simulink model "gm_mpu6050_interfaceasdf"  (R2017a)
settings: Solver=FixedStepDiscrete  StartTime=0.0  StopTime=inf  RelTol=1e-3  EnableMultiTasking=on
PostLoadFcn:
  | ChipSelect = 1;  % choose I2C comms
  | AddressAlt = 0;  % use default address
  | 
  | if AddressAlt == 1
  | % b1101001 (pin AD0 is logic high).
  | SlvAddr = uint8(bin2dec('1101001'));  % ADDR ALT = 1
  | else
  | % b1101000 (pin AD0 is logic low)
  | SlvAddr = uint8(bin2dec('1101000'));  % ADDR ALT = 0
  | end
  | SlvAddr = uint8(hex2dec('68'));
  | 
  | 
  | % 0x3B 59 ACCEL_XOUT[15:8]
  | % 0x3C 60 ACCEL_XOUT[7:0]
  | % 0x3D 61 ACCEL_YOUT[15:8]
  | % 0x3E 62 ACCEL_YOUT[7:0]
  | % 0x3F 63 ACCEL_ZOUT[15:8]
  | % 0x40 64 ACCEL_ZOUT[7:0]
  | 
  | AccelXRegAddr = uint8(hex2dec('3B'));
  | AccelYRegAddr = uint8(hex2dec('3D'));
  | AccelZRegAddr = uint8(hex2dec('3F'));
  | 
  | % 0x43 67 GYRO_XOUT[15:8]
  | % 0x44 68 GYRO_XOUT[7:0]
  | % 0x45 69 GYRO_YOUT[15:8]
  | % 0x46 70 GYRO_YOUT[7:0]
  | % 0x47 71 GYRO_ZOUT[15:8]
  | % 0x48 72 GYRO_ZOUT[7:0]
  | 
  | GyroXRegAddr = uint8(hex2dec('43'));
  | GyroYRegAddr = uint8(hex2dec('45'));
  | GyroZRegAddr = uint8(hex2dec('47'));
  | 
  | deviceAddr = fi(SlvAddr,0,7,0);
  | 
  | powerRegAddr = uint8(hex2dec('6B'));
  | powerRegData = bin2dec('10000001');
undefined symbols (not defined in the file): AXI4, Lite
libraries: axiinterfacelib x10
settings Model: SimulationMode=external  Creator=skuznick  LastModifiedBy=mini
settings SolverCC: EnableConcurrentExecution=on  ConcurrentTasks=on  PositivePriorityOrder=on
settings DataIOCC: SaveOutput=off  SaveTime=off
settings OptimizationCC: BlockReduction=off  ConditionallyExecuteInputs=off  PassReuseOutputArgsAs=Individual arguments  MaxStackSize=64
settings DebuggingCC: AlgebraicLoopMsg=error  SingleTaskRateTransMsg=error  ParameterTunabilityLossMsg=error
settings HardwareCC: ProdBitPerPointer=32  ProdBitPerSizeT=32  ProdBitPerPtrDiffT=32  ProdLargestAtomicInteger=Long  ProdLargestAtomicFloat=Double  ProdWordSize=32  ProdHWDeviceType=ARM Compatible->ARM Cortex  TargetEndianess=LittleEndian
settings SFSimCC: MATLABDynamicMemAlloc=off
settings RTWCC: SystemTargetFile=ert.tlc  HardwareBoard=ZedBoard  TLCOptions="-aInlineSetEventsForThisBaseRateFcn=TLC_FALSE -aSuppressMultiTaskScheduler=TLC_FALSE  -aRateBasedStepFcn=0"  TemplateMakefile=ert_default_tmf  Description=Embedded Coder  GenerateReport=on  Toolchain=Xilinx Software Development Kit (SDK)  IncludeHyperlinkInReport=on  LaunchReport=on  GenerateTraceInfo=on  GenerateTraceReport=on  GenerateTraceReportSl=on  GenerateTraceReportSf=on  GenerateTraceReportEml=on
settings CodeAppCC: ForceParamTrailComments=on  IgnoreCustomStorageClasses=off  OperatorAnnotations=on  SimulinkDataObjDesc=on  SFDataObjDesc=on  MATLABFcnDesc=on  InsertBlockDesc=on  MATLABSourceComments=on

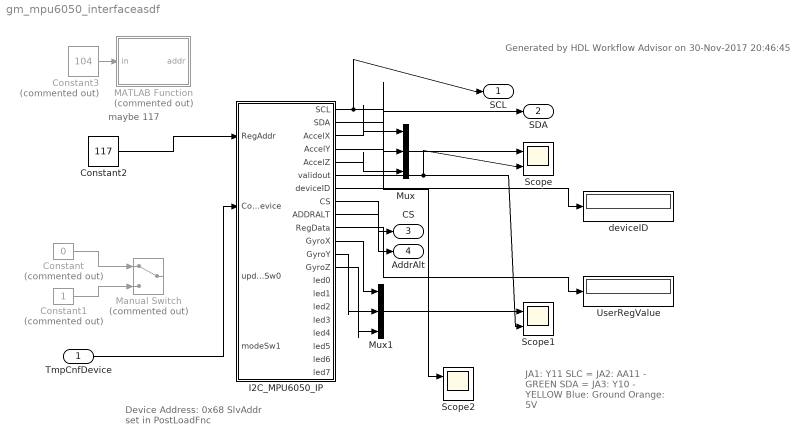
== system gm_mpu6050_interfaceasdf ==
  note: Device Address: 0x68
      | SlvAddr set in PostLoadFnc
  note: JA1: Y11
      | SLC = JA2: AA11 - GREEN
      | SDA = JA3: Y10  - YELLOW
      | Blue: Ground
      | Orange: 5V
  note: maybe 117
  note: Generated by HDL Workflow Advisor on 30-Nov-2017 20:46:45
  TmpCnfDevice : Inport  OutDataTypeStr=boolean
  Constant : Constant  Commented=on  Value=0  OutDataTypeStr=boolean  SampleTime=-1
  Constant1 : Constant  Commented=on  OutDataTypeStr=boolean  SampleTime=-1
  Constant2 : Constant  Value=117  OutDataTypeStr=uint8  SampleTime=-1
  Constant3 : Constant  Commented=on  Value=104  OutDataTypeStr=uint8  SampleTime=-1
  I2C_MPU6050_IP : Subsystem  TreatAsAtomicUnit=on  mask(AXI4-Lite/AXI4 Interface){}
      mask help:
      | This is an automatically generated subsystem block.
      | This contains the AXI interface blocks that communicate with the ADXL345_ip IPCore generated from mpu6050/I2C_MPU6050_IP subsystem.
      mask Display: disp(sprintf('Xilinx Zynq \nAXI Interface'));
  MATLAB Function : MATLAB Function  Commented=on  TreatAsAtomicUnit=on
  Manual Switch : ManualSwitch  Commented=on
  Mux : Mux  Inputs=3
  Mux1 : Mux  Inputs=3
  Scope : Scope  NumInputPorts=2
  Scope1 : Scope  NumInputPorts=2
  Scope2 : Scope  NumInputPorts=2
  UserRegValue : Display
  deviceID : Display
  SCL : Outport
  SDA : Outport  Port=2
  CS : Outport  Port=3
  AddrAlt : Outport  Port=4
  wires:
  Constant3/1 -> MATLAB Function/1(in)
  TmpCnfDevice/1 -> I2C_MPU6050_IP/2(ConfigDevice)
  I2C_MPU6050_IP/6(validout) -> Scope1/2, Scope/2
  I2C_MPU6050_IP/12(GyroY) -> Mux1/2
  I2C_MPU6050_IP/11(GyroX) -> Mux1/1
  I2C_MPU6050_IP/13(GyroZ) -> Mux1/3
  Mux1/1 -> Scope1/1
  Constant2/1 -> I2C_MPU6050_IP/1(RegAddr)
  Constant1/1 -> Manual Switch/2
  Constant/1 -> Manual Switch/1
  Mux/1 -> Scope/1
  I2C_MPU6050_IP/10(RegData) -> UserRegValue/1
  I2C_MPU6050_IP/7(deviceID) -> deviceID/1
  I2C_MPU6050_IP/5(AccelZ) -> Mux/3
  I2C_MPU6050_IP/3(AccelX) -> Mux/1
  I2C_MPU6050_IP/4(AccelY) -> Mux/2
  I2C_MPU6050_IP/9(ADDRALT) -> AddrAlt/1
  I2C_MPU6050_IP/8(CS) -> CS/1
  I2C_MPU6050_IP/1(SCL) -> SCL/1, Scope2/1
  I2C_MPU6050_IP/2(SDA) -> SDA/1

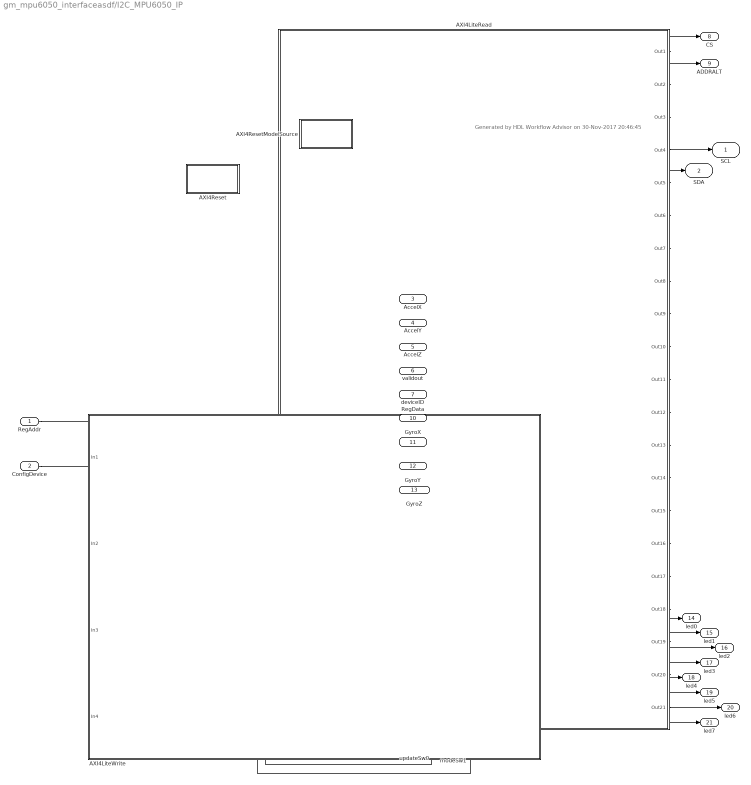
== system gm_mpu6050_interfaceasdf/I2C_MPU6050_IP ==
  note: Generated by HDL Workflow Advisor on 30-Nov-2017 20:46:45
  RegAddr : Inport
  ConfigDevice : Inport  Port=2
  updateSw0 : Inport  Port=3  OutDataTypeStr=boolean
  modeSw1 : Inport  Port=4  OutDataTypeStr=boolean
  AXI4LiteRead : Subsystem  Priority=10
  AXI4LiteWrite : Subsystem  Priority=1
  AXI4Reset : Subsystem  mask(System Start){ShowInLibBrowser=0}
      mask prompts: ShowInLibBrowser "Simulink:masks:CustCodeMaskParam1_MP"
      settings: CopyFcn=cccopyfcn(gcb)  OpenFcn=ccopenfcn('System Start Function')
      mask Help: eval('feval(''rtwprivate'',''rtwhelpview'',''rtw_sys_start_block'')');
      mask Display: disp('System\nStart');
  AXI4ResetModelSource : Subsystem  mask(Model Source){ShowInLibBrowser=0}
      mask prompts: ShowInLibBrowser "Simulink:masks:CustCodeMaskParam1_MP"
      settings: CopyFcn=cccopyfcn(gcb)  OpenFcn=ccopenfcn('Model Source')
      mask Help: eval('feval(''rtwprivate'',''rtwhelpview'',''rtw_model_source_block'')');
      mask Display: disp('Model\nSource');
  SCL : Outport
  SDA : Outport  Port=2
  AccelX : Outport  Port=3
  AccelY : Outport  Port=4
  AccelZ : Outport  Port=5
  validout : Outport  Port=6
  deviceID : Outport  Port=7
  CS : Outport  Port=8
  ADDRALT : Outport  Port=9
  RegData : Outport  Port=10
  GyroX : Outport  Port=11
  GyroY : Outport  Port=12
  GyroZ : Outport  Port=13
  led0 : Outport  Port=14  OutDataTypeStr=boolean
  led1 : Outport  Port=15  OutDataTypeStr=boolean
  led2 : Outport  Port=16  OutDataTypeStr=boolean
  led3 : Outport  Port=17  OutDataTypeStr=boolean
  led4 : Outport  Port=18  OutDataTypeStr=boolean
  led5 : Outport  Port=19  OutDataTypeStr=boolean
  led6 : Outport  Port=20  OutDataTypeStr=boolean
  led7 : Outport  Port=21  OutDataTypeStr=boolean
  wires:
  RegAddr/1 -> AXI4LiteWrite/1(In1)
  ConfigDevice/1 -> AXI4LiteWrite/2(In2)
  updateSw0/1 -> AXI4LiteWrite/3(In3)
  modeSw1/1 -> AXI4LiteWrite/4(In4)
  AXI4LiteRead/1(Out1) -> CS/1
  AXI4LiteRead/2(Out2) -> ADDRALT/1
  AXI4LiteRead/3(Out3) -> SCL/1
  AXI4LiteRead/4(Out4) -> SDA/1
  AXI4LiteRead/5(Out5) -> AccelX/1
  AXI4LiteRead/6(Out6) -> AccelY/1
  AXI4LiteRead/7(Out7) -> AccelZ/1
  AXI4LiteRead/8(Out8) -> validout/1
  AXI4LiteRead/9(Out9) -> deviceID/1
  AXI4LiteRead/10(Out10) -> RegData/1
  AXI4LiteRead/11(Out11) -> GyroX/1
  AXI4LiteRead/12(Out12) -> GyroY/1
  AXI4LiteRead/13(Out13) -> GyroZ/1
  AXI4LiteRead/14(Out14) -> led0/1
  AXI4LiteRead/15(Out15) -> led1/1
  AXI4LiteRead/16(Out16) -> led2/1
  AXI4LiteRead/17(Out17) -> led3/1
  AXI4LiteRead/18(Out18) -> led4/1
  AXI4LiteRead/19(Out19) -> led5/1
  AXI4LiteRead/20(Out20) -> led6/1
  AXI4LiteRead/21(Out21) -> led7/1

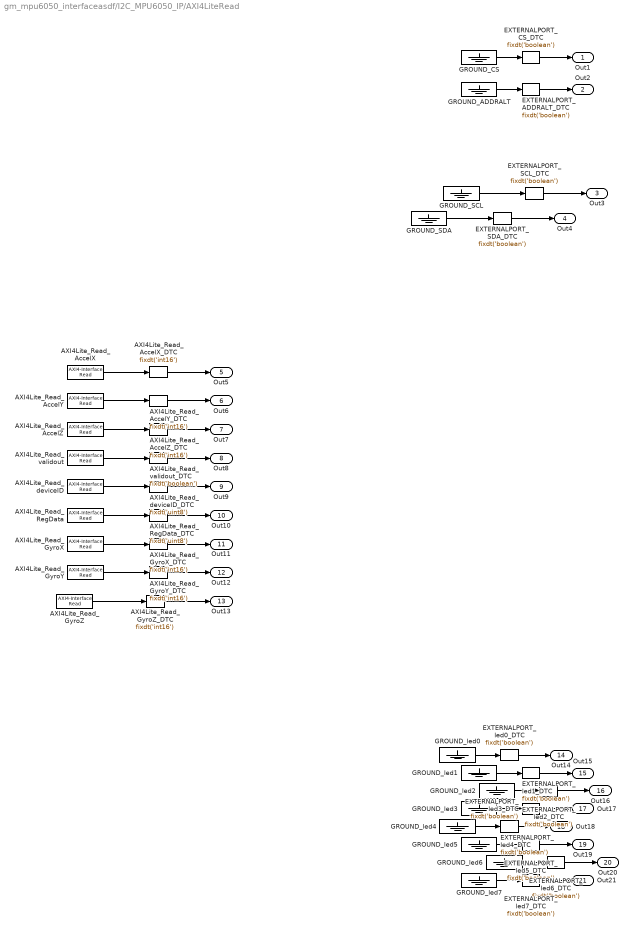
== system gm_mpu6050_interfaceasdf/I2C_MPU6050_IP/AXI4LiteRead ==
  AXI4Lite_Read_AccelX : axiinterfacelib/AXI4-Interface Read  Priority=4  AXIInterfaceType=AXI4-Lite  DeviceName=/dev/mwipcore  RegisterOffset=hex2dec('108')  DataLength=1  DataType=uint32  SampleTime=-1  blockPlatform=ZYNQ  SimulateUsing=Interpreted Execution
      settings: SourceProductName=Embedded Coder Support Package for Xilinx Zynq-7000 Platform  SourceProductBaseCode=ECZYNQ7000
  AXI4Lite_Read_AccelX_DTC : DataTypeConversion  OutDataTypeStr=fixdt('int16')  ConvertRealWorld=Stored Integer (SI)
  AXI4Lite_Read_AccelY : axiinterfacelib/AXI4-Interface Read  Priority=5  AXIInterfaceType=AXI4-Lite  DeviceName=/dev/mwipcore  RegisterOffset=hex2dec('10C')  DataLength=1  DataType=uint32  SampleTime=-1  blockPlatform=ZYNQ  SimulateUsing=Interpreted Execution
      settings: SourceProductName=Embedded Coder Support Package for Xilinx Zynq-7000 Platform  SourceProductBaseCode=ECZYNQ7000
  AXI4Lite_Read_AccelY_DTC : DataTypeConversion  OutDataTypeStr=fixdt('int16')  ConvertRealWorld=Stored Integer (SI)
  AXI4Lite_Read_AccelZ : axiinterfacelib/AXI4-Interface Read  Priority=6  AXIInterfaceType=AXI4-Lite  DeviceName=/dev/mwipcore  RegisterOffset=hex2dec('110')  DataLength=1  DataType=uint32  SampleTime=-1  blockPlatform=ZYNQ  SimulateUsing=Interpreted Execution
      settings: SourceProductName=Embedded Coder Support Package for Xilinx Zynq-7000 Platform  SourceProductBaseCode=ECZYNQ7000
  AXI4Lite_Read_AccelZ_DTC : DataTypeConversion  OutDataTypeStr=fixdt('int16')  ConvertRealWorld=Stored Integer (SI)
  AXI4Lite_Read_GyroX : axiinterfacelib/AXI4-Interface Read  Priority=12  AXIInterfaceType=AXI4-Lite  DeviceName=/dev/mwipcore  RegisterOffset=hex2dec('124')  DataLength=1  DataType=uint32  SampleTime=-1  blockPlatform=ZYNQ  SimulateUsing=Interpreted Execution
      settings: SourceProductName=Embedded Coder Support Package for Xilinx Zynq-7000 Platform  SourceProductBaseCode=ECZYNQ7000
  AXI4Lite_Read_GyroX_DTC : DataTypeConversion  OutDataTypeStr=fixdt('int16')  ConvertRealWorld=Stored Integer (SI)
  AXI4Lite_Read_GyroY : axiinterfacelib/AXI4-Interface Read  Priority=13  AXIInterfaceType=AXI4-Lite  DeviceName=/dev/mwipcore  RegisterOffset=hex2dec('128')  DataLength=1  DataType=uint32  SampleTime=-1  blockPlatform=ZYNQ  SimulateUsing=Interpreted Execution
      settings: SourceProductName=Embedded Coder Support Package for Xilinx Zynq-7000 Platform  SourceProductBaseCode=ECZYNQ7000
  AXI4Lite_Read_GyroY_DTC : DataTypeConversion  OutDataTypeStr=fixdt('int16')  ConvertRealWorld=Stored Integer (SI)
  AXI4Lite_Read_GyroZ : axiinterfacelib/AXI4-Interface Read  Priority=14  AXIInterfaceType=AXI4-Lite  DeviceName=/dev/mwipcore  RegisterOffset=hex2dec('12C')  DataLength=1  DataType=uint32  SampleTime=-1  blockPlatform=ZYNQ  SimulateUsing=Interpreted Execution
      settings: SourceProductName=Embedded Coder Support Package for Xilinx Zynq-7000 Platform  SourceProductBaseCode=ECZYNQ7000
  AXI4Lite_Read_GyroZ_DTC : DataTypeConversion  OutDataTypeStr=fixdt('int16')  ConvertRealWorld=Stored Integer (SI)
  AXI4Lite_Read_RegData : axiinterfacelib/AXI4-Interface Read  Priority=11  AXIInterfaceType=AXI4-Lite  DeviceName=/dev/mwipcore  RegisterOffset=hex2dec('120')  DataLength=1  DataType=uint32  SampleTime=-1  blockPlatform=ZYNQ  SimulateUsing=Interpreted Execution
      settings: SourceProductName=Embedded Coder Support Package for Xilinx Zynq-7000 Platform  SourceProductBaseCode=ECZYNQ7000
  AXI4Lite_Read_RegData_DTC : DataTypeConversion  OutDataTypeStr=fixdt('uint8')  ConvertRealWorld=Stored Integer (SI)
  AXI4Lite_Read_deviceID : axiinterfacelib/AXI4-Interface Read  Priority=8  AXIInterfaceType=AXI4-Lite  DeviceName=/dev/mwipcore  RegisterOffset=hex2dec('11C')  DataLength=1  DataType=uint32  SampleTime=-1  blockPlatform=ZYNQ  SimulateUsing=Interpreted Execution
      settings: SourceProductName=Embedded Coder Support Package for Xilinx Zynq-7000 Platform  SourceProductBaseCode=ECZYNQ7000
  AXI4Lite_Read_deviceID_DTC : DataTypeConversion  OutDataTypeStr=fixdt('uint8')  ConvertRealWorld=Stored Integer (SI)
  AXI4Lite_Read_validout : axiinterfacelib/AXI4-Interface Read  Priority=7  AXIInterfaceType=AXI4-Lite  DeviceName=/dev/mwipcore  RegisterOffset=hex2dec('118')  DataLength=1  DataType=uint32  SampleTime=-1  blockPlatform=ZYNQ  SimulateUsing=Interpreted Execution
      settings: SourceProductName=Embedded Coder Support Package for Xilinx Zynq-7000 Platform  SourceProductBaseCode=ECZYNQ7000
  AXI4Lite_Read_validout_DTC : DataTypeConversion  OutDataTypeStr=fixdt('boolean')  ConvertRealWorld=Stored Integer (SI)
  EXTERNALPORT_ADDRALT_DTC : DataTypeConversion  OutDataTypeStr=fixdt('boolean')
  EXTERNALPORT_CS_DTC : DataTypeConversion  OutDataTypeStr=fixdt('boolean')
  EXTERNALPORT_SCL_DTC : DataTypeConversion  OutDataTypeStr=fixdt('boolean')
  EXTERNALPORT_SDA_DTC : DataTypeConversion  OutDataTypeStr=fixdt('boolean')
  EXTERNALPORT_led0_DTC : DataTypeConversion  OutDataTypeStr=fixdt('boolean')
  EXTERNALPORT_led1_DTC : DataTypeConversion  OutDataTypeStr=fixdt('boolean')
  EXTERNALPORT_led2_DTC : DataTypeConversion  OutDataTypeStr=fixdt('boolean')
  EXTERNALPORT_led3_DTC : DataTypeConversion  OutDataTypeStr=fixdt('boolean')
  EXTERNALPORT_led4_DTC : DataTypeConversion  OutDataTypeStr=fixdt('boolean')
  EXTERNALPORT_led5_DTC : DataTypeConversion  OutDataTypeStr=fixdt('boolean')
  EXTERNALPORT_led6_DTC : DataTypeConversion  OutDataTypeStr=fixdt('boolean')
  EXTERNALPORT_led7_DTC : DataTypeConversion  OutDataTypeStr=fixdt('boolean')
  GROUND_ADDRALT : Ground
  GROUND_CS : Ground
  GROUND_SCL : Ground
  GROUND_SDA : Ground
  GROUND_led{0..7} (8 alike) : Ground
  Out1 : Outport
  Out2 : Outport  Port=2
  Out3 : Outport  Port=3
  Out4 : Outport  Port=4
  Out5 : Outport  Port=5
  Out6 : Outport  Port=6
  Out7 : Outport  Port=7
  Out8 : Outport  Port=8
  Out9 : Outport  Port=9
  Out10 : Outport  Port=10
  Out11 : Outport  Port=11
  Out12 : Outport  Port=12
  Out13 : Outport  Port=13
  Out14 : Outport  Port=14
  Out15 : Outport  Port=15
  Out16 : Outport  Port=16
  Out17 : Outport  Port=17
  Out18 : Outport  Port=18
  Out19 : Outport  Port=19
  Out20 : Outport  Port=20
  Out21 : Outport  Port=21
  wires:
  AXI4Lite_Read_RegData/1 -> AXI4Lite_Read_RegData_DTC/1
  AXI4Lite_Read_RegData_DTC/1 -> Out10/1
  AXI4Lite_Read_GyroX/1 -> AXI4Lite_Read_GyroX_DTC/1
  AXI4Lite_Read_GyroX_DTC/1 -> Out11/1
  GROUND_led0/1 -> EXTERNALPORT_led0_DTC/1
  AXI4Lite_Read_GyroZ/1 -> AXI4Lite_Read_GyroZ_DTC/1
  AXI4Lite_Read_GyroZ_DTC/1 -> Out13/1
  GROUND_led1/1 -> EXTERNALPORT_led1_DTC/1
  EXTERNALPORT_led1_DTC/1 -> Out15/1
  EXTERNALPORT_led0_DTC/1 -> Out14/1
  GROUND_led2/1 -> EXTERNALPORT_led2_DTC/1
  EXTERNALPORT_led4_DTC/1 -> Out18/1
  GROUND_led3/1 -> EXTERNALPORT_led3_DTC/1
  EXTERNALPORT_led2_DTC/1 -> Out16/1
  GROUND_led4/1 -> EXTERNALPORT_led4_DTC/1
  EXTERNALPORT_led3_DTC/1 -> Out17/1
  GROUND_led5/1 -> EXTERNALPORT_led5_DTC/1
  EXTERNALPORT_led5_DTC/1 -> Out19/1
  GROUND_led6/1 -> EXTERNALPORT_led6_DTC/1
  EXTERNALPORT_led6_DTC/1 -> Out20/1
  GROUND_led7/1 -> EXTERNALPORT_led7_DTC/1
  EXTERNALPORT_led7_DTC/1 -> Out21/1
  AXI4Lite_Read_AccelZ/1 -> AXI4Lite_Read_AccelZ_DTC/1
  AXI4Lite_Read_AccelZ_DTC/1 -> Out7/1
  AXI4Lite_Read_GyroY/1 -> AXI4Lite_Read_GyroY_DTC/1
  AXI4Lite_Read_GyroY_DTC/1 -> Out12/1
  EXTERNALPORT_CS_DTC/1 -> Out1/1
  AXI4Lite_Read_deviceID_DTC/1 -> Out9/1
  GROUND_CS/1 -> EXTERNALPORT_CS_DTC/1
  GROUND_ADDRALT/1 -> EXTERNALPORT_ADDRALT_DTC/1
  EXTERNALPORT_ADDRALT_DTC/1 -> Out2/1
  EXTERNALPORT_SCL_DTC/1 -> Out3/1
  GROUND_SDA/1 -> EXTERNALPORT_SDA_DTC/1
  GROUND_SCL/1 -> EXTERNALPORT_SCL_DTC/1
  EXTERNALPORT_SDA_DTC/1 -> Out4/1
  AXI4Lite_Read_AccelX/1 -> AXI4Lite_Read_AccelX_DTC/1
  AXI4Lite_Read_AccelX_DTC/1 -> Out5/1
  AXI4Lite_Read_validout_DTC/1 -> Out8/1
  AXI4Lite_Read_deviceID/1 -> AXI4Lite_Read_deviceID_DTC/1
  AXI4Lite_Read_AccelY_DTC/1 -> Out6/1
  AXI4Lite_Read_validout/1 -> AXI4Lite_Read_validout_DTC/1
  AXI4Lite_Read_AccelY/1 -> AXI4Lite_Read_AccelY_DTC/1

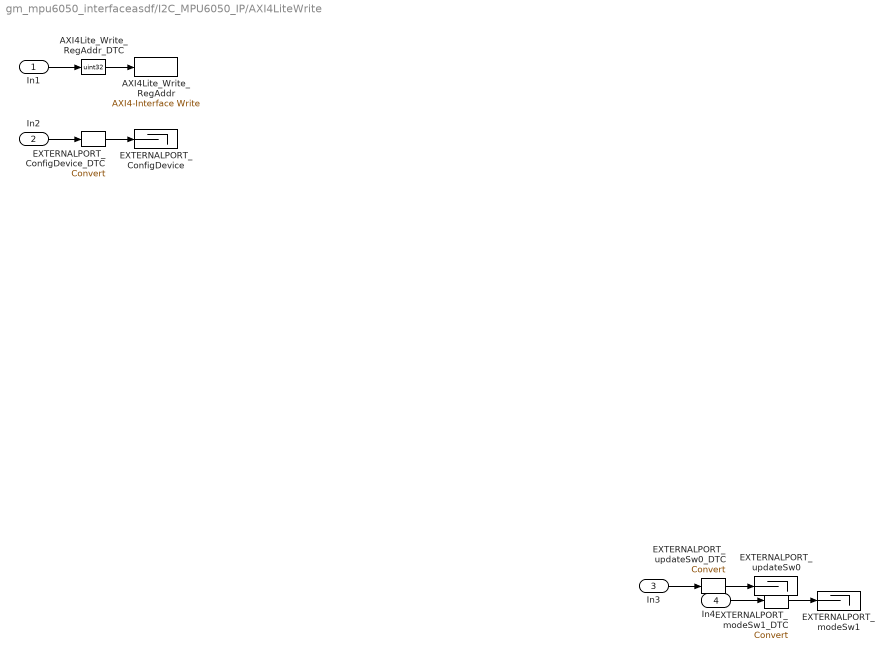
== system gm_mpu6050_interfaceasdf/I2C_MPU6050_IP/AXI4LiteWrite ==
  In1 : Inport
  In2 : Inport  Port=2
  In3 : Inport  Port=3
  In4 : Inport  Port=4
  AXI4Lite_Write_RegAddr : axiinterfacelib/AXI4-Interface Write  Priority=1  AXIInterfaceType=AXI4-Lite  DeviceName=/dev/mwipcore  RegisterOffset=hex2dec('114')  blockPlatform=ZYNQ  SimulateUsing=Interpreted execution
      settings: SourceProductName=Embedded Coder Support Package for Xilinx Zynq-7000 Platform  SourceProductBaseCode=ECZYNQ7000
  AXI4Lite_Write_RegAddr_DTC : DataTypeConversion  OutDataTypeStr=uint32  ConvertRealWorld=Stored Integer (SI)
  EXTERNALPORT_ConfigDevice : Terminator
  EXTERNALPORT_ConfigDevice_DTC : DataTypeConversion
  EXTERNALPORT_modeSw1 : Terminator
  EXTERNALPORT_modeSw1_DTC : DataTypeConversion
  EXTERNALPORT_updateSw0 : Terminator
  EXTERNALPORT_updateSw0_DTC : DataTypeConversion
  wires:
  In1/1 -> AXI4Lite_Write_RegAddr_DTC/1
  EXTERNALPORT_ConfigDevice_DTC/1 -> EXTERNALPORT_ConfigDevice/1
  EXTERNALPORT_modeSw1_DTC/1 -> EXTERNALPORT_modeSw1/1
  In2/1 -> EXTERNALPORT_ConfigDevice_DTC/1
  EXTERNALPORT_updateSw0_DTC/1 -> EXTERNALPORT_updateSw0/1
  In4/1 -> EXTERNALPORT_modeSw1_DTC/1
  AXI4Lite_Write_RegAddr_DTC/1 -> AXI4Lite_Write_RegAddr/1
  In3/1 -> EXTERNALPORT_updateSw0_DTC/1

== system gm_mpu6050_interfaceasdf/I2C_MPU6050_IP/AXI4Reset ==

== system gm_mpu6050_interfaceasdf/I2C_MPU6050_IP/AXI4ResetModelSource ==

== matlab function gm_mpu6050_interfaceasdf/MATLAB Function ==
  data: in input; addr output
function addr = fcn(in)
    addr = uint8(in);
